simulink model "speed_control_of_bldc_motor_for_variable_speed"  (R2019a)
settings: Solver=ode3  StartTime=0.0  StopTime=13  RelTol=1e-3
libraries: powerlib x9, simulink x9
settings Model: Creator=Deepak  LastModifiedBy=Deepak
settings DebuggingCC: ArithmeticOperatorsInVariantConditions=warning
settings CodeAppCC: StateflowObjectComments=on

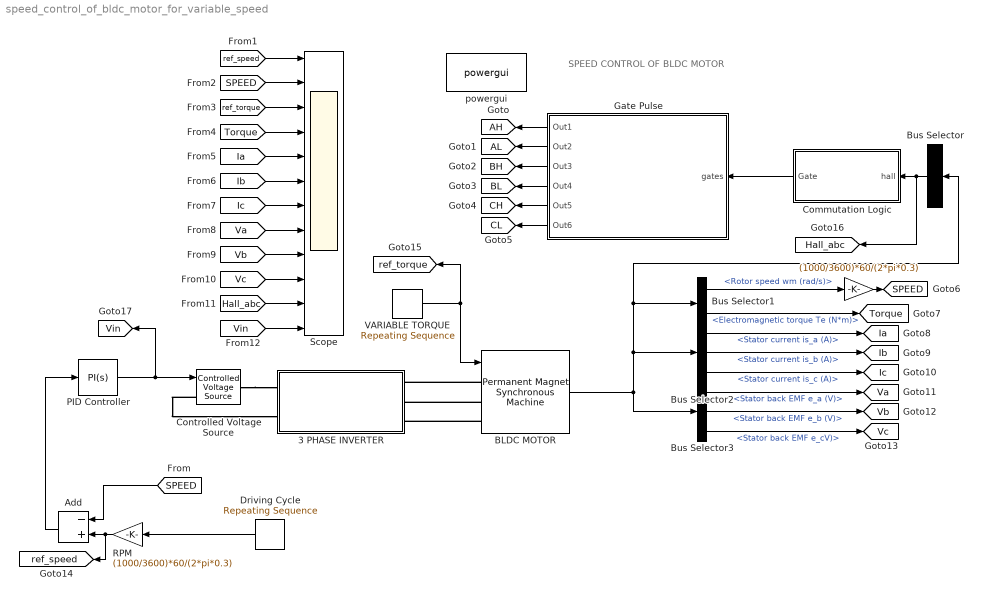
== system speed_control_of_bldc_motor_for_variable_speed ==
  note: SPEED CONTROL OF BLDC MOTOR
  " " : Gain  Gain=(1000/3600)*60/(2*pi*0.3)
  " RPM" : Gain  Gain=(1000/3600)*60/(2*pi*0.3)
  3 PHASE INVERTER : Subsystem
  Add : Sum  Inputs=-+
  BLDC MOTOR : powerlib/Machines/Permanent Magnet Synchronous Machine  NbPhases=3  FluxDistribution=Trapezoidal  RotorType=Round  MechanicalLoad=Torque Tm  PresetModel=No  ShowDetailedParameters=on  MeasurementBus=off  Resistance=0.7  Inductance=2.7e-3  dqInductances=[8.5e-3,8.5e-3]  La=0.000395  MachineConstant=Flux linkage established by magnets (V.s)  Flux=0.1194  VoltageCst=100.0283  TorqueCst=0.9552  Flat=120  Mechanical=[0.0027 0.0004924 4 0]  PolePairs=4  InitialConditions=[0,0, 0,0]  InitialConditions5ph=[0 0 0 0 0 0]  TsPowergui=0  TsBlock=-1  RefAngle=90 degrees behind phase A axis (modified Park)
  Bus Selector : BusSelector  OutputSignals=Hall effect signal h_a,Hall effect signal h_b,Hall effect signal h_c  OutputAsBus=on
  Bus Selector1 : BusSelector  OutputSignals=Rotor speed wm (rad/s),Electromagnetic torque Te (N*m)
  Bus Selector2 : BusSelector  OutputSignals=Stator current is_a (A),Stator current is_b (A),Stator current is_c (A)
  Bus Selector3 : BusSelector  OutputSignals=Stator back EMF e_a (V),Stator back EMF e_b (V),Stator back EMF e_cV)
  Commutation Logic : Subsystem
  Controlled Voltage Source : powerlib/Electrical Sources/Controlled Voltage Source  Initialize=on  Source_Type=DC  Amplitude=160  Phase=0  Frequency=0  Measurements=None
      settings: SourceProductName=Simscape Electrical
  Driving Cycle : simulink/Sources/Repeating Sequence  rep_seq_t=[0 1 2 3 4 5 6 7 8 9 10 11 11.0001 12 13]  rep_seq_y=[0 0 20 20 0 0 30 30 0 0 50 50 40 40 0]
  Gate Pulse : Subsystem
  PID Controller : simulink/Continuous/PID Controller  Controller=PI  Form=Parallel  TimeDomain=Continuous-time  SampleTime=-1  IntegratorMethod=Forward Euler  FilterMethod=Forward Euler  ControllerParametersSource=internal  P=0.754336715688095  I=49.9879440674314  D=0.00192762182262476  UseFilter=on  N=289.099868323626  TunerSelectOption=Transfer Function Based (PID Tuner App)  InitialConditionSource=internal  InitialConditionForIntegrator=0  InitialConditionForFilter=0  DifferentiatorICPrevScaledInput=0  ExternalReset=none  TrackingMode=off  Kt=1  LimitOutput=off  UpperSaturationLimit=inf  LowerSaturationLimit=-inf  LinearizeAsGain=on  AntiWindupMode=none  Kb=1  POutMin=[]  POutMax=[]  IOutMin=[]  IOutMax=[]  DOutMin=[]  DOutMax=[]  NOutMin=[]  NOutMax=[]  SumOutMin=[]  SumOutMax=[]  SaturationOutMin=[]  SaturationOutMax=[]  PParamMin=[]  PParamMax=[]  IParamMin=[]  IParamMax=[]  DParamMin=[]  DParamMax=[]  NParamMin=[]  NParamMax=[]  KbParamMin=[]  KbParamMax=[]  KtParamMin=[]  KtParamMax=[]  KbOutMin=[]  KbOutMax=[]  KtOutMin=[]  KtOutMax=[]  IntegratorOutMin=[]  IntegratorOutMax=[]  FilterOutMin=[]  FilterOutMax=[]  SumI1OutMin=[]  SumI1OutMax=[]  SumI2OutMin=[]  SumI2OutMax=[]  SumI3OutMin=[]  SumI3OutMax=[]  SumI4OutMin=[]  SumI4OutMax=[]  SumDOutMin=[]  SumDOutMax=[]  DifferentiatorOutMin=[]  DifferentiatorOutMax=[]  FilterDiffOutCoefMin=[]  FilterDiffOutCoefMax=[]  ReciprocalOutMin=[]  ReciprocalOutMax=[]  SumDenOutMin=[]  SumDenOutMax=[]  SumNumOutMin=[]  SumNumOutMax=[]  DivideOutMin=[]  DivideOutMax=[]  IntegratorContinuousStateAttributes=''  IntegratorStateMustResolveToSignalObject=off  IntegratorRTWStateStorageClass=Auto  FilterContinuousStateAttributes=''  FilterStateMustResolveToSignalObject=off  FilterRTWStateStorageClass=Auto  ParallelPVariant=InternalParameters  IdealPVariant=Disabled  IVariant=InternalParameters  DVariant=Disabled  IntegratorVariant=Continuous  SatVariant=Disabled  AWVariant=Passthrough  PCopyVariant=Disabled  TRVariant=Disabled  FdbkBlocksVariant=Forward  IdealPFdbkVariant=Disabled  SatFdbkVariant=Disabled  DerivativeFilterVariant=Disabled  NVariant=Disabled  NCopyVariant=Disabled_SignalSpec  FilterICVariant=Disabled  IntegratorICVariant=InternalICs  ExternalResetVariant=Disabled  TRSumVariant=Passthrough  SumFdbkVariant=Disabled  SumVariant=Sum_PI
  Scope : Scope  NumInputPorts=12
  VARIABLE TORQUE : simulink/Sources/Repeating Sequence  rep_seq_t=[0 1 2 3 4 5 6 7 8 9 10 11 12 13]  rep_seq_y=[3 3 3 3 5 5 5 -2 -2 -2 1 1 1 1 ]
  powergui : powerlib/powergui  Priority=1  SimulationMode=Discrete  SampleTime=50e-6  frequency=60  Iterations=50  frequencyindice=0  Pbase=100e6  ErrMax=1e-4  UnitsV=kV  UnitsW=MW  buscounter=0  FunctionMessages=off  echomessages=off  EnableUseOfTLC=off  CurrentSourceSwitches=off  DisableSnubberDevices=off  DisableRonSwitches=off  DisableVfSwitches=off  DisplayEquations=off  AutomaticDiscreteSolvers=off  SolverType=Tustin/Backward Euler (TBE)  Interpol=off  ExternalGateDelay=off  methode=off  Ts=100  x0status=blocks  SPID=on  SwTol=0  HookPort=off  NonlinearTolerance=0  nMaxIteration=15  ContinueOnMaxIteration=off  RestoreLinks=warning  ResistiveCurrentMeasurement=off  Frange=[0:2:500]  Ylog=off  Xlog=on  ShowGrid=off  save=off  variable=ZData  structure=0  ZoomFFT=off  StartTime=0.0  cycles=1  DisplayStyle=1  fundamental=60  FreqAxis=off  MaxFrequency=1000  frequencyindicesteady=1  RmsSteady=1  display=off
      settings: SourceProductName=Simscape Electrical
  tag scope: AH=global, AL=global, BH=global, BL=global, CH=global, CL=global, Hall_abc=global, Ia=global, Ib=global, Ic=global, SPEED=global, Torque=global, Va=global, Vb=global, Vc=global, Vin=global, ref_speed=global, ref_torque=global
  wires:
  Commutation Logic/1(Gate) -> Gate Pulse/1(gates)
  VARIABLE TORQUE/1 -> BLDC MOTOR/1, [ref_torque]
  BLDC MOTOR/1 -> Bus Selector3/1, Bus Selector/1, Bus Selector1/1, Bus Selector2/1
  PID Controller/1 -> [Vin], Controlled Voltage Source/1
  Add/1 -> PID Controller/1
  " RPM"/1 -> [ref_speed], Add/2
  Gate Pulse/1(Out1) -> [AH]
  Gate Pulse/2(Out2) -> [AL]
  Gate Pulse/3(Out3) -> [BH]
  Gate Pulse/4(Out4) -> [BL]
  Gate Pulse/5(Out5) -> [CH]
  Gate Pulse/6(Out6) -> [CL]
  Bus Selector/1 -> [Hall_abc], Commutation Logic/1("hall ")
  Bus Selector1/2 -> [Torque]  "<Electromagnetic torque Te (N*m)>"
  Bus Selector2/1 -> [Ia]  "<Stator current is_a (A)>"
  Bus Selector2/2 -> [Ib]  "<Stator current is_b (A)>"
  Bus Selector2/3 -> [Ic]  "<Stator current is_c (A)>"
  Bus Selector3/1 -> [Va]  "<Stator back EMF e_a (V)>"
  Bus Selector3/2 -> [Vb]  "<Stator back EMF e_b (V)>"
  Bus Selector3/3 -> [Vc]  "<Stator back EMF e_cV)>"
  [SPEED] -> Add/1
  Bus Selector1/1 -> " "/1  "<Rotor speed wm (rad/s)>"
  " "/1 -> [SPEED]
  [ref_speed] -> Scope/1
  [SPEED] -> Scope/2
  [ref_torque] -> Scope/3
  [Torque] -> Scope/4
  [Ia] -> Scope/5
  [Ib] -> Scope/6
  [Ic] -> Scope/7
  [Va] -> Scope/8
  [Vb] -> Scope/9
  [Vc] -> Scope/10
  [Hall_abc] -> Scope/11
  [Vin] -> Scope/12
  Driving Cycle/1 -> " RPM"/1
  connections:
  BLDC MOTOR/LConn1 -- 3 PHASE INVERTER/RConn1
  BLDC MOTOR/LConn2 -- 3 PHASE INVERTER/RConn2
  BLDC MOTOR/LConn3 -- 3 PHASE INVERTER/RConn3
  Controlled Voltage Source/RConn1 -- 3 PHASE INVERTER/LConn1
  Controlled Voltage Source/LConn1 -- 3 PHASE INVERTER/LConn2

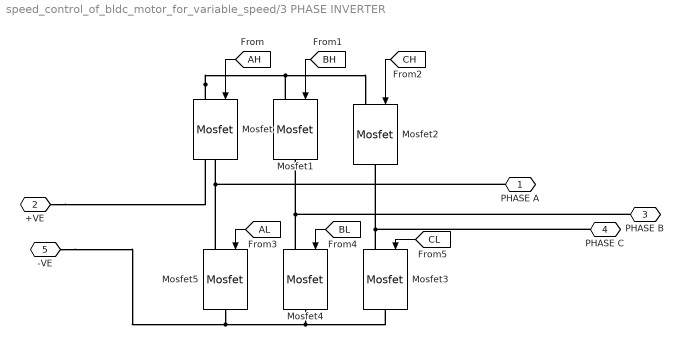
== system speed_control_of_bldc_motor_for_variable_speed/3 PHASE INVERTER ==
  Mosfet{,1..5} (6 alike) : powerlib/Power Electronics/Mosfet  Ron=0.1  Lon=0  Rd=0.01  Vfd=0  IC=0  Rs=1e5  Cs=inf  Measurements=off
      settings: SourceProductName=Simscape Electrical
  PHASE A : PMIOPort  Side=Right
  +VE : PMIOPort  Port=2  Side=Left
  PHASE B : PMIOPort  Port=3  Side=Right
  PHASE C : PMIOPort  Port=4  Side=Right
  -VE : PMIOPort  Port=5  Side=Left
  wires:
  [AH] -> Mosfet/1
  [BH] -> Mosfet1/1
  [CH] -> Mosfet2/1
  [AL] -> Mosfet5/1
  [BL] -> Mosfet4/1
  [CL] -> Mosfet3/1
  connections:
  Mosfet5/LConn1 -- Mosfet/RConn1 -- PHASE A/RConn1
  Mosfet4/LConn1 -- Mosfet1/RConn1 -- PHASE B/RConn1
  Mosfet3/LConn1 -- PHASE C/RConn1 -- Mosfet2/RConn1
  Mosfet/LConn1 -- Mosfet1/LConn1 -- Mosfet2/LConn1 -- +VE/RConn1
  Mosfet5/RConn1 -- -VE/RConn1 -- Mosfet4/RConn1 -- Mosfet3/RConn1

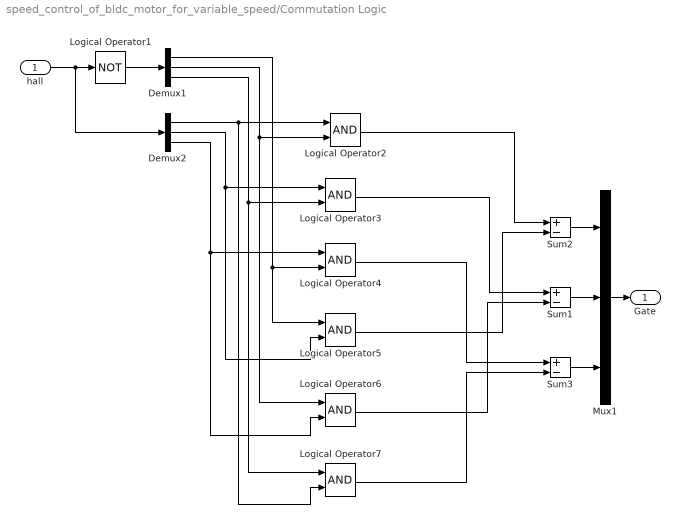
== system speed_control_of_bldc_motor_for_variable_speed/Commutation Logic ==
  "hall " : Inport
  Demux1 : Demux  Outputs=3
  Demux2 : Demux  Outputs=3
  Logical Operator1 : Logic  Operator=NOT  AllPortsSameDT=off  OutDataTypeStr=boolean
  Logical Operator{2..7} (6 alike) : Logic  AllPortsSameDT=off  OutDataTypeStr=boolean
  Mux1 : Mux  Inputs=3
  Sum1 : Sum  Inputs=+-  OutDataTypeStr=double
  Sum2 : Sum  Inputs=+-  OutDataTypeStr=double
  Sum3 : Sum  Inputs=+-  OutDataTypeStr=double
  Gate : Outport
  wires:
  Demux2/1 -> Logical Operator7/2, Logical Operator2/1
  Demux1/3 -> Logical Operator7/1, Logical Operator3/2
  Demux2/2 -> Logical Operator3/1, Logical Operator5/2
  Sum1/1 -> Mux1/2
  Logical Operator3/1 -> Sum1/1
  "hall "/1 -> Logical Operator1/1, Demux2/1
  Demux1/2 -> Logical Operator6/1, Logical Operator2/2
  Logical Operator2/1 -> Sum2/1
  Logical Operator7/1 -> Sum3/2
  Logical Operator4/1 -> Sum3/1
  Demux1/1 -> Logical Operator4/2, Logical Operator5/1
  Logical Operator6/1 -> Sum1/2
  Logical Operator5/1 -> Sum2/2
  Sum3/1 -> Mux1/3
  Logical Operator1/1 -> Demux1/1
  Mux1/1 -> Gate/1
  Sum2/1 -> Mux1/1
  Demux2/3 -> Logical Operator4/1, Logical Operator6/2

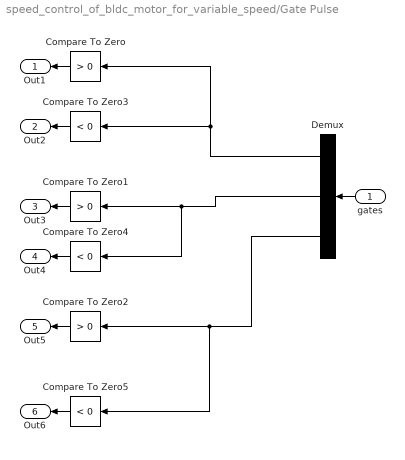
== system speed_control_of_bldc_motor_for_variable_speed/Gate Pulse ==
  gates : Inport
  Compare To Zero : simulink/Logic and Bit Operations/Compare To Zero  relop=>  OutDataTypeStr=boolean
  Compare To Zero1 : simulink/Logic and Bit Operations/Compare To Zero  relop=>  OutDataTypeStr=boolean
  Compare To Zero2 : simulink/Logic and Bit Operations/Compare To Zero  relop=>  OutDataTypeStr=boolean
  Compare To Zero3 : simulink/Logic and Bit Operations/Compare To Zero  relop=<  OutDataTypeStr=boolean
  Compare To Zero4 : simulink/Logic and Bit Operations/Compare To Zero  relop=<  OutDataTypeStr=boolean
  Compare To Zero5 : simulink/Logic and Bit Operations/Compare To Zero  relop=<  OutDataTypeStr=boolean
  Demux : Demux  Outputs=3
  Out1 : Outport
  Out2 : Outport  Port=2
  Out3 : Outport  Port=3
  Out4 : Outport  Port=4
  Out5 : Outport  Port=5
  Out6 : Outport  Port=6
  wires:
  Compare To Zero1/1 -> Out3/1
  Demux/2 -> Compare To Zero4/1, Compare To Zero1/1
  Compare To Zero3/1 -> Out2/1
  Demux/3 -> Compare To Zero5/1, Compare To Zero2/1
  Compare To Zero2/1 -> Out5/1
  Demux/1 -> Compare To Zero3/1, Compare To Zero/1
  Compare To Zero4/1 -> Out4/1
  Compare To Zero5/1 -> Out6/1
  Compare To Zero/1 -> Out1/1
  gates/1 -> Demux/1
